simulink model "PID_Regler2test_vers5"  (Simulink 7.6)
settings: Solver=ode45  SolverMode=SingleTasking  StartTime=0.0  StopTime=100000  RelTol=1e-3
libraries: simulink x1, modelsimlib x1, simulink_extras x1
settings Model: Creator=azafar  LastModifiedBy=localadmin
settings OptimizationCC: InlineParams=on
settings DebuggingCC: FcnCallInpInsideContextMsg=Enable All
settings HardwareCC: ProdHWDeviceType=ASIC/FPGA->ASIC/FPGA  TargetIntDivRoundTo=Zero  TargetEndianess=LittleEndian  TargetHWDeviceType=MATLAB Host  ProdEqTarget=off

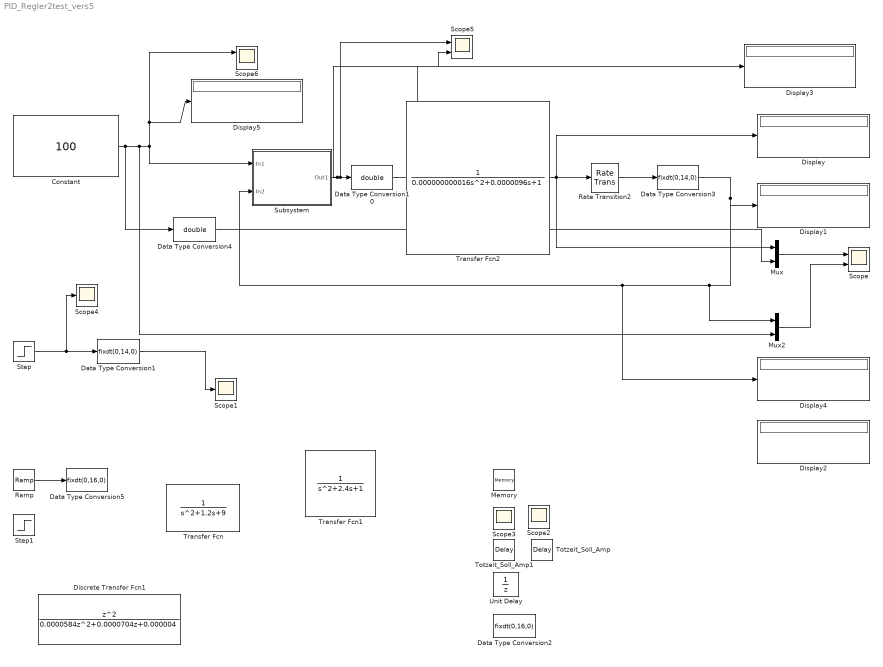
== system PID_Regler2test_vers5 ==
  Constant : Constant  Value=100  OutDataTypeStr=fixdt(0,14,0)  SampleTime=1
  Data Type Conversion1 : DataTypeConversion  OutDataTypeStr=fixdt(0,14,0)  SampleTime=1
  Data Type Conversion10 : DataTypeConversion  OutDataTypeStr=double  SampleTime=1
  Data Type Conversion2 : DataTypeConversion  OutDataTypeStr=fixdt(0,16,0)  SampleTime=1
  Data Type Conversion3 : DataTypeConversion  OutDataTypeStr=fixdt(0,14,0)  SampleTime=1
  Data Type Conversion4 : DataTypeConversion  OutDataTypeStr=double  SampleTime=1
  Data Type Conversion5 : DataTypeConversion  OutDataTypeStr=fixdt(0,16,0)  SampleTime=1
  Discrete Transfer Fcn1 : DiscreteTransferFcn  Numerator=[1 0 0]  Denominator=[0.0000584 0.0000704 0.000004]  StateDataTypeStr=int16
  Display{,1..5} (6 alike) : Display
      Display settings: Format=decimal (Stored Integer)
      Display1 settings: Format=decimal (Stored Integer)
      Display2 settings: Format=binary (Stored Integer)
      Display3 settings: Format=decimal (Stored Integer)
      Display4 settings: Format=binary (Stored Integer)
      Display5 settings: Format=decimal (Stored Integer)
  Memory : Memory
  Mux : Mux  Inputs=2
  Mux2 : Mux  Inputs=2
  Ramp : simulink/Sources/Ramp  SystemSampleTime=-1  slope=1  start=1  X0=0
  Rate Transition2 : RateTransition  OutPortSampleTime=1
  Scope{,2,5..6} (4 alike) : Scope  NumInputPorts=2
      Scope settings: TimeRange=0.018  YMin=7703.389830508476~0  YMax=8073.849878934626~600
      Scope2 settings: YMin=9.5~9.5  YMax=10.5~10.5  SaveName=ScopeData4
      Scope5 settings: TimeRange=35  YMin=23502~23502  YMax=23503~23503  SaveName=ScopeData8
      Scope6 settings: TimeRange=10000  YMin=0.95~-5  YMax=1.05~5  SaveName=ScopeData9
  Scope1 : Scope
      settings: TimeRange=10000  YMin=0.95  YMax=1.05  SaveName=ScopeData3
  Scope3 : Scope
      settings: SaveName=ScopeData5
  Scope4 : Scope
      settings: TimeRange=10000  YMin=0.95  YMax=1.05  SaveName=ScopeData6
  Step : Step  Time=0.0001  Before=1  SampleTime=1
  Step1 : Step  Time=0.0001  Before=1  After=2  SampleTime=1
  Subsystem : Subsystem
  Totzeit_Soll_Amp : TransportDelay  DelayTime=0.5*10^(-5)
  Totzeit_Soll_Amp1 : TransportDelay  DelayTime=0.5*10^(-5)
  Transfer Fcn : TransferFcn  Denominator=[1 1.2 9]
  Transfer Fcn1 : TransferFcn  Denominator=[1 2.4 1]
  Transfer Fcn2 : TransferFcn  Denominator=[0.000000000016 0.0000096 1]
  Unit Delay : UnitDelay  SampleTime=-1
  wires:
  Mux/1 -> Scope/1
  Subsystem/1(Out1) -> Scope5/1, Data Type Conversion10/1, Display3/1
  Transfer Fcn2/1 -> Mux/1, Display/1, Rate Transition2/1
  Data Type Conversion10/1 -> Scope5/2, Transfer Fcn2/1
  Data Type Conversion3/1 -> Display1/1, Subsystem/2(In2), Display4/1, Mux2/1
  Data Type Conversion1/1 -> Scope1/1
  Constant/1 -> Data Type Conversion4/1, Display5/1, Scope6/1, Subsystem/1(In1), Mux2/2
  Step/1 -> Scope4/1, Data Type Conversion1/1
  Ramp/1 -> Data Type Conversion5/1
  Mux2/1 -> Scope/2
  Data Type Conversion4/1 -> Mux/2
  Rate Transition2/1 -> Data Type Conversion3/1

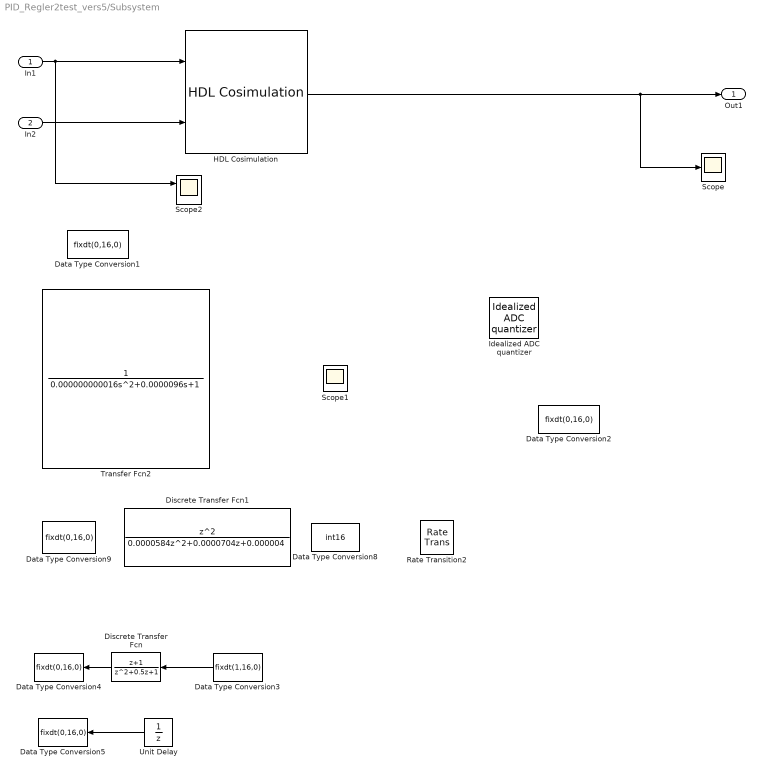
== system PID_Regler2test_vers5/Subsystem ==
  In1 : Inport  OutDataTypeStr=fixdt(0,14,0)
  In2 : Inport  Port=2  OutDataTypeStr=fixdt(0,14,0)
  Data Type Conversion1 : DataTypeConversion  OutDataTypeStr=fixdt(0,16,0)
  Data Type Conversion{2,4..5,9} (4 alike) : DataTypeConversion  OutDataTypeStr=fixdt(0,16,0)  SampleTime=1
  Data Type Conversion3 : DataTypeConversion  OutDataTypeStr=fixdt(1,16,0)  SampleTime=1
  Data Type Conversion8 : DataTypeConversion  OutDataTypeStr=int16  SampleTime=1
  Discrete Transfer Fcn : DiscreteTransferFcn  Numerator=[1 1]  Denominator=[1 0.5 1]  StateDataTypeStr=fixdt(1,16,0)
  Discrete Transfer Fcn1 : DiscreteTransferFcn  Numerator=[1 0 0]  Denominator=[0.0000584 0.0000704 0.000004]  StateDataTypeStr=fixdt(1,16,0)
  HDL Cosimulation : modelsimlib/HDL Cosimulation  DialogController=hdllinkddg.CoSimBlockDialog  SystemSampleTime=-1  PortPaths=/pi_controller_and_feed_forward_tb/dut/data_w_i;/pi_controller_and_feed_forward_tb/dut/data_y_i;/pi_controller_and_feed_forward_tb/dut/data_u_o  PortModes=[1 1 2 ]  PortTimes=[-1,-1,10]  PortSigns=[-1 -1 -1 ]  PortFracLengths=[0,0,0]  CommLocal=on  CommSharedMemory=on  CommPortNumber=4449  CommShowInfo=on  ClockPaths=/pi_controller_and_feed_forward_tb/dut/clk_i  ClockModes=[2 ]  ClockTimes=[2]  TclPreSimCommand="echo \"Running pi_controller_and_feed_forward in Simulink.\""  TclPostSimCommand="echo \"Done\""  TimingMode=s  TimingScaleFactor=1e-012  idxCellArray={'UNUSED_VAR'}  CosimBypass=Full Simulation  AllowDirectFeedthrough=on  ProductName=EDA Simulator Link MQ  RunAutoTimescale=off  HdlClocks=0
      link override Inport__pi_controller_and_feed_forward_tb_dut_data_w_i: Port=1
  Idealized ADC quantizer : simulink_extras/Additional Discrete/Idealized ADC quantizer  SystemSampleTime=-1  NumberOfConverterBits=16  Vmin=0  Vmax=1  OutputDataType=uint16  OutputNegativeValues=off
  Rate Transition2 : RateTransition  OutPortSampleTime=1
  Scope : Scope
      settings: TimeRange=627.563576702215  YMin=18500  YMax=19550
  Scope1 : Scope
      settings: TimeRange=100  YMin=0  YMax=70000  SaveName=ScopeData2
  Scope2 : Scope  NumInputPorts=2
      settings: TimeRange=5000  YMin=0~13106  YMax=2~13108  SaveName=ScopeData7
  Transfer Fcn2 : TransferFcn  Denominator=[0.000000000016 0.0000096 1]
  Unit Delay : UnitDelay
  Out1 : Outport  OutDataTypeStr=fixdt(0,14,0)
  wires:
  In1/1 -> Scope2/1, HDL Cosimulation/1
  HDL Cosimulation/1 -> Out1/1, Scope/1
  Discrete Transfer Fcn/1 -> Data Type Conversion4/1
  Data Type Conversion3/1 -> Discrete Transfer Fcn/1
  Unit Delay/1 -> Data Type Conversion5/1
  In2/1 -> HDL Cosimulation/2
